simulink model "PTDLHN_2020a"  (R2020a)
settings: Solver=VariableStepAuto  StartTime=0.0  StopTime=10.0  RelTol=1e-3
settings Model: Creator=Hp  LastModifiedBy=Hp
settings DebuggingCC: SFMachineParentedDataDiag=error

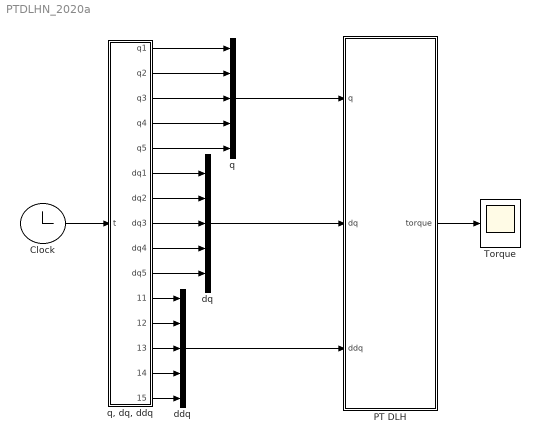
== system PTDLHN_2020a ==
  Clock : Clock
  PT DLH : MATLAB Function  TreatAsAtomicUnit=on
  Torque : Scope
  ddq : Mux  Inputs=5
  dq : Mux  Inputs=5
  "q " : Mux  Inputs=5
  "q, dq, ddq" : MATLAB Function  TreatAsAtomicUnit=on
  wires:
  Clock/1 -> "q, dq, ddq"/1(t)
  "q, dq, ddq"/1(q1) -> "q "/1
  "q, dq, ddq"/2(q2) -> "q "/2
  "q, dq, ddq"/3(q3) -> "q "/3
  "q, dq, ddq"/4(q4) -> "q "/4
  "q, dq, ddq"/5(q5) -> "q "/5
  "q, dq, ddq"/6(dq1) -> dq/1
  "q, dq, ddq"/7(dq2) -> dq/2
  "q, dq, ddq"/8(dq3) -> dq/3
  "q, dq, ddq"/9(dq4) -> dq/4
  "q, dq, ddq"/10(dq5) -> dq/5
  "q, dq, ddq"/11(ddq1) -> ddq/1
  "q, dq, ddq"/12(ddq2) -> ddq/2
  "q, dq, ddq"/13(ddq3) -> ddq/3
  "q, dq, ddq"/14(ddq4) -> ddq/4
  "q, dq, ddq"/15(ddq5) -> ddq/5
  "q "/1 -> PT DLH/1(q)
  dq/1 -> PT DLH/2(dq)
  ddq/1 -> PT DLH/3(ddq)
  PT DLH/1(torque) -> Torque/1

== matlab function PTDLHN_2020a/PT DLH ==
  data: q input; dq input; torque output; ddq input
function torque = fcn(q, dq, ddq)
L1=2; % m
L2=2;
a2=1;
L3=1.5;
L4=1;
L5=0.75;

m2=2;
m3=1;
m4=0.75;
m5=0.5;

I2x=10^(-4);
I2y=10^(-4);
I2z=10^(-4);

I3x=10^(-4);
I3y=10^(-4);
I3z=10^(-4);

I4x=10^(-4);
I4y=10^(-4);
I4z=10^(-4);

I5x=10^(-4);
I5y=10^(-4);
I5z=10^(-4);
%Ma tran M
M=zeros(5,5);
M(1,1)= m2 + m3 + m4 + m5;
M(1,2)= -((m5 * (2 * L4 + L5) + m4 * L4) * cos(q(4)) + (2 * a2 * (m3 + m4 + m5))) * sin(q(2)) / 0.2e1;
M(1,3)= 0;
M(1,4)= -sin(q(4)) * cos(q(2)) * ((m4 + 2 * m5) * L4 + m5 * L5) / 0.2e1;
M(1,5)= 0;

M(2,1)= -((m5 * (2 * L4 + L5) + m4 * L4) * cos(q(4)) + (2 * a2 * (m3 + m4 + m5))) * sin(q(2)) / 0.2e1;
M(2,2)= ((-4 * I5x + 4 * I5y) * cos(q(5)) ^ 2 + 0.4e1 * (L4 + L5 / 0.2e1) ^ 2 * m5 + m4 * L4 ^ 2 - (4 * I4x) + (4 * I4y) + (4 * I5x) - (4 * I5z)) * cos(q(4)) ^ 2 / 0.4e1 + (m5 * (0.2e1 * L4 + L5) + m4 * L4) * a2 * cos(q(4)) + ((4 * m3) + 0.4e1 * m4 + 0.4e1 * m5) * a2 ^ 2 / 0.4e1 + I3z + I4x + I5z + I2z;
M(2,3)= 0;
M(2,4)= sin(q(5)) * cos(q(5)) * cos(q(4)) * (I5x - I5y);
M(2,5)= -sin(q(4)) * I5z;

M(3,1)= 0;
M(3,2)= 0;
M(3,3)= m3 + m4 + m5;
M(3,4)= -((m4 + 2 * m5) * L4 + m5 * L5) * cos(q(4)) / 0.2e1;
M(3,5)= 0;

M(4,1)= -sin(q(4)) * cos(q(2)) * ((m4 + 2 * m5) * L4 + m5 * L5) / 0.2e1;
M(4,2)= sin(q(5)) * cos(q(5)) * cos(q(4)) * (I5x - I5y);
M(4,3)= -((m4 + 2 * m5) * L4 + m5 * L5) * cos(q(4)) / 0.2e1;
M(4,4)= m4 * L4 ^ 2 / 0.4e1 + I4z + (I5x - I5y) * cos(q(5)) ^ 2 + (0.2e1 * L4 + L5) ^ 2 * m5 / 0.4e1 + I5y;
M(4,5)= 0;

M(5,1)= 0;
M(5,2)= -sin(q(4)) * I5z;
M(5,3)= 0;
M(5,4)= 0;
M(5,5)= I5z

%Ma tran C
C=zeros(5,5);
C(1,1)= 0;
C(1,2)= -((m5 * (2 * L4 + L5) + m4 * L4) * cos(q(4)) + (2 * a2 * (m3 + m4 + m5))) * cos(q(2)) * dq(2) / 0.2e1 + sin(q(4)) * (m5 * (2 * L4 + L5) + m4 * L4) * sin(q(2)) * dq(4) / 0.2e1;
C(1,3)= 0;
C(1,4)= -(dq(4) * cos(q(2)) * cos(q(4)) - dq(2) * sin(q(2)) * sin(q(4))) * ((m4 + 2 * m5) * L4 + m5 * L5) / 0.2e1;
C(1,5)= 0;

C(2,1)= -((m5 * (2 * L4 + L5) + m4 * L4) * cos(q(4)) + (2 * a2 * (m3 + m4 + m5))) * cos(q(2)) * dq(2) / 0.4e1 + sin(q(4)) * (m5 * (2 * L4 + L5) + m4 * L4) * sin(q(2)) * dq(4) / 0.4e1;
C(2,2)= 0.2e1 * dq(5) * cos(q(5)) * sin(q(5)) * (I5x - I5y) * cos(q(4)) ^ 2 + (-0.2e1 * dq(4) * ((-0.4e1 * I5x + 0.4e1 * I5y) * cos(q(5)) ^ 2 + 0.4e1 * (L4 + L5 / 0.2e1) ^ 2 * m5 + m4 * L4 ^ 2 - (4 * I4x) + (4 * I4y) + 0.4e1 * I5x - (4 * I5z)) * sin(q(4)) + cos(q(2)) * (m5 * (0.2e1 * L4 + L5) + m4 * L4) * dq(1)) * cos(q(4)) / 0.4e1 - a2 * (dq(4) * (m5 * (0.2e1 * L4 + L5) + m4 * L4) * sin(q(4)) - dq(1) * cos(q(2)) * (m3 + m4 + m5) / 0.2e1);
C(2,3)= 0;
C(2,4)=  (-0.4e1 * (I5x - I5y) * cos(q(5)) * sin(q(5)) * dq(4) - ((m4 + 2 * m5) * L4 + m5 * L5) * dq(1) * sin(q(2))) * sin(q(4)) / 0.4e1 + 0.2e1 * (I5x - I5y) * cos(q(4)) * (cos(q(5)) ^ 2 - 0.1e1 / 0.2e1) * dq(5);
C(2,5)= -I5z * cos(q(4)) * dq(4);

C(3,1)= 0;
C(3,2)= 0;
C(3,3)= 0;
C(3,4)=((m4 + 2 * m5) * L4 + m5 * L5) * sin(q(4)) * dq(4) / 0.2e1;
C(3,5)= 0;

C(4,1)= -(dq(4) * cos(q(2)) * cos(q(4)) - dq(2) * sin(q(2)) * sin(q(4))) * ((m4 + 2 * m5) * L4 + m5 * L5) / 0.4e1;
C(4,2)= (((-4 * I5x + 4 * I5y) * cos(q(5)) ^ 2 + ((m4 + 4 * m5) * L4 ^ 2) + (4 * L4 * L5 * m5) + (L5 ^ 2 * m5) + (4 * I5x) - (4 * I5z) - (4 * I4x) + (4 * I4y)) * dq(2) * cos(q(4)) - 0.2e1 * (I5x - I5y) * cos(q(5)) * sin(q(5)) * dq(4) - (dq(1) * sin(q(2)) - 0.2e1 * dq(2) * a2) * ((m4 + 2 * m5) * L4 + m5 * L5)) * sin(q(4)) / 0.4e1 + 0.2e1 * cos(q(4)) * dq(5) * ((I5x - I5y) * cos(q(5)) ^ 2 - I5x / 0.2e1 + I5y / 0.2e1 + I5z / 0.4e1);
C(4,3)= ((m4 + 2 * m5) * L4 + m5 * L5) * sin(q(4)) * dq(4) / 0.4e1;
C(4,4)= (0.2e1 * dq(2) * sin(q(5)) * (I5x - I5y) * cos(q(5)) - (((m4 + 2 * m5) * L4 + m5 * L5) * dq(3))) * sin(q(4)) / 0.4e1 - 0.2e1 * (I5x - I5y) * cos(q(5)) * sin(q(5)) * dq(5) + cos(q(4)) * cos(q(2)) * ((m4 + 2 * m5) * L4 + m5 * L5) * dq(1) / 0.4e1;
C(4,5)= I5z * cos(q(4)) * dq(2) / 0.2e1;

C(5,1)= 0;
C(5,2)= -cos(q(4)) * (dq(4) * (I5x - I5y) * cos(q(5)) ^ 2 + sin(q(5)) * dq(2) * cos(q(4)) * (I5x - I5y) * cos(q(5)) - dq(4) * (I5x - I5y - (2 * I5z)) / 0.2e1);
C(5,3)= 0;
C(5,4)= -(I5x - I5y) * (dq(2) * (cos(q(5)) ^ 2 - 0.1e1 / 0.2e1) * cos(q(4)) - cos(q(5)) * sin(q(5)) * dq(4));
C(5,5)= 0;

%Ma tran G
G=zeros(5,1);
G(1,1)= 0;
G(2,1)= 0;
G(3,1)= 10*(m3 + m4);
G(4,1)= -5*m4*L4*cos(q(4));
G(5,1)= 0;

torque = M*ddq + C*dq + G;

== matlab function PTDLHN_2020a/q, dq, ddq ==
  data: t input; q1 output; q2 output; q3 output; q4 output; q5 output; dq1 output; dq2 output; dq3 output; dq4 output; dq5 output; ddq1 output; ddq2 output; ddq3 output; ddq4 output; ddq5 output
function [q1,q2,q3,q4,q5,dq1,dq2,dq3,dq4,dq5,ddq1,ddq2,ddq3,ddq4,ddq5] = fcn(t)
q1=sin(t)+1;
q2=pi*cos(t);
q3=0.75*(cos(t)+1);
q4=-(pi/6)*cos(t)-(pi/2);
q5=pi*sin(t)

dq1=cos(t);
dq2=-pi*sin(t);
dq3=-0.75*sin(t);
dq4=(pi/6)*sin(t);
dq5=pi*cos(t)

ddq1=-sin(t);
ddq2=-pi*cos(t);
ddq3=-0.75*cos(t);
ddq4=(pi/6)*cos(t);
ddq5=-pi*sin(t)
end
